simulink model "Diode"  (R2020b)
settings: Solver=FixedStepAuto  StartTime=0.0  StopTime=10.0  RelTol=1e-3
model workspace (MAT data in the model file):
  CurrentmA = Simulink.Parameter
  CurrentmA.Value = [0; 0; 5; 10; 15; 20; 25; 30; 35; 40; 45; 50; 55; 60; 65; 70; 75; 80; 85; 90; 95; 100]
  CurrentmA.DataType = 'auto'
  CurrentmA.Dimensions = [22 1]
  ForwardVoltagev = Simulink.Parameter
  ForwardVoltagev.Value = [0; 0.58; 0.66; 0.69; 0.7; 0.71; 0.72; 0.73; 0.74; 0.74; 0.75; 0.75; 0.75; 0.76; 0.76; 0.76; 0.77; 0.77; 0.77; 0.77; 0.77; 0.77]
  ForwardVoltagev.DataType = 'auto'
  ForwardVoltagev.Dimensions = [22 1]
  data = Simulink.Parameter
  data.Value = [0; 0.58; 0.69; 0.72; 0.75; 0.77]
  data.DataType = 'auto'
  data.Dimensions = [6 1]
libraries: simulink x1
settings Model: OrderedModelArguments=off  Creator=Administrator  LastModifiedBy=Administrator

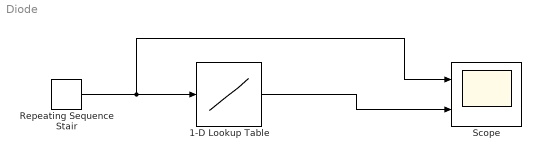
== system Diode ==
  1-D Lookup Table : Lookup_n-D  NumberOfTableDimensions=1  BreakpointsForDimension1=CurrentmA  Table=ForwardVoltagev  InternalRulePriority=Speed  RndMeth=Simplest  InputSameDT=on
  Repeating Sequence Stair : simulink/Sources/Repeating Sequence Stair  OutValues=data  tsamp=-1  OutMin=[]  OutMax=[]  OutDataTypeStr=double  OutputDataTypeScalingMode=double  OutDataType=fixdt(0,8)  ConRadixGroup=Best Precision: Vector-wise  OutScaling=2^-12
  Scope : Scope  NumInputPorts=2
  wires:
  Repeating Sequence Stair/1 -> Scope/1, 1-D Lookup Table/1
  1-D Lookup Table/1 -> Scope/2
